simulink model "oculomotor_fb_HW1_2b"  (Simulink 7.8)
settings: Solver=ode45  SolverMode=SingleTasking  StartTime=0.0  StopTime=10  RelTol=1e-3  AbsTol=1e-6
settings Model: Creator=sschaal  LastModifiedBy=okhan  ExtModeAutoUpdateStatusClock=off
settings DataIOCC: LimitDataPoints=off  SaveOutput=off  SaveTime=off  SignalLoggingName=sigsOut
settings OptimizationCC: BooleanDataType=off  InlineInvariantSignals=on  InitFltsAndDblsToZero=on
settings DebuggingCC: SaveWithParameterizedLinksMsg=none  SignalResolutionControl=TryResolveAllWithWarning  SolverPrmCheckMsg=none  MultiTaskDSMMsg=warning  MultiTaskCondExecSysMsg=none  FcnCallInpInsideContextMsg=Use local settings  StrictBusMsg=None
settings HardwareCC: TargetUnknown=on
settings RTWCC: IncludeERTFirstTime=on
settings GRTTargetCC: TargetFcnLib=ansi_tfl_tmw.mat  ModelReferenceCompliant=off  MatFileLogging=off

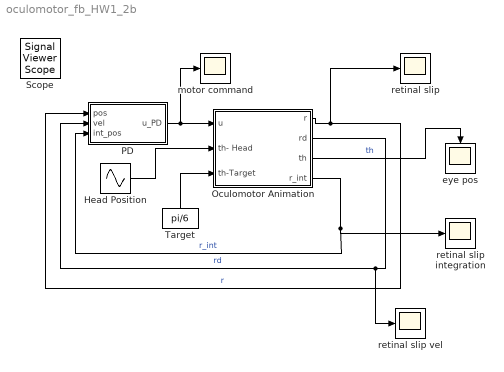
== system oculomotor_fb_HW1_2b ==
  " Target" : Constant  Value=pi/6
  Head Position : Sin  Amplitude=pi/6  Frequency=6  SampleTime=0
  Oculomotor Animation : Subsystem  mask(Oculomotor Animation){ts=0.6, delay=2/60*0.0000001, k=0.4875, b=0.0341, m=3.6889e-4}
      mask prompts: ts "Animation Sampling Time (ts)"; delay "Retinal Slip Delay (delay)"; k "Stiffness (k)"; b "Damping (b)"; m "Mass (m)"
      mask help:
      | Animation Sampling Time: at which freq. to redraw of the animation
      | x-offset: horizontal offset of eye rotation axis from head rotation axis
      | y-offset: vertical offset of eye rotation axis from head rotation axis
      | slip & slip vel. delays: simulated delays for slip computation
      | mass, damping, stiffness: parameters of eye system
      mask Help:
      | Implementation of a second order dynamical model of a 2-eye oculomotor system. Input to the system are the motor commands for left and right eye,
      | the head movement (cause by neck movement or external perturbations), the angle of the visual target (in world coord.), and the foveal length.
      | Outputs are the retinal slip & slip vel. for both eyes and the eye positions.
  PD : Subsystem  mask(PID Controller){P=20, D=0.05, I=1000}
      mask prompts: P "Proportional (P):"; D "Derivative (D):"; I "Integral (I):"
      mask help:
      | Enter expressions for proportional and derivative terms.
      | P+Ds
      mask Help: This block implements a PD controller where parameters are entered for the Proportional and Derivative terms. Unmask this block to see how it works.
  eye pos : Scope
      settings: TickLabels=on  YMin=-0.2  YMax=0.2  DataFormat=Array
  motor command : Scope
      settings: TickLabels=on  YMin=-1  YMax=1  DataFormat=Array
  retinal slip : Scope
      settings: TickLabels=on  TimeRange=10  YMin=0  YMax=0.55  DataFormat=Array
  retinal slip integration : Scope
      settings: TickLabels=on  YMin=-0.2  YMax=0.2  DataFormat=Array
  retinal slip vel : Scope
      settings: TickLabels=on  YMin=-0.2  YMax=0.2  DataFormat=Array
  Scope : SignalViewerScope  IOType=viewer  ZoomMode=xonly  LegendLocations="552.963      402.4925       78.0331      32.50355"  RefreshTime=0.035000
      settings: ShowLegends=on  TimeRange=10  YMin=-0.2  YMax=1.2
  wires:
  " Target"/1 -> Oculomotor Animation/3(th-Target)
  Head Position/1 -> Oculomotor Animation/2(th- Head)
  PD/1(u_PD) -> motor command/1, Oculomotor Animation/1(u)
  Oculomotor Animation/1(r) -> retinal slip/1, PD/1(pos)  "r"
  Oculomotor Animation/2(rd) -> PD/2(vel), retinal slip vel/1  "rd"
  Oculomotor Animation/3(th) -> eye pos/1  "th"
  Oculomotor Animation/4(r_int) -> PD/3(int_pos), retinal slip integration/1  "r_int"

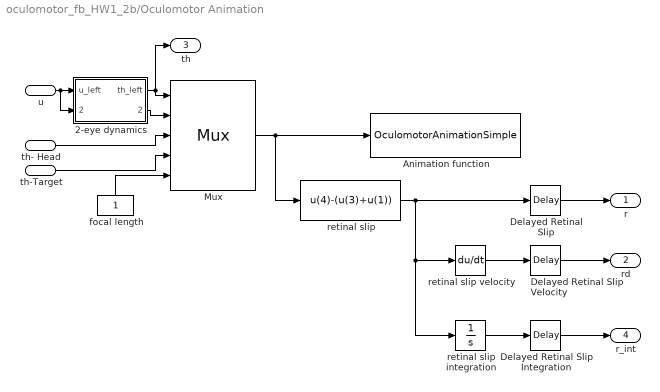
== system oculomotor_fb_HW1_2b/Oculomotor Animation ==
  u : Inport
  th- Head : Inport  Port=2
  th-Target : Inport  Port=3
  " focal length" : Constant
  2-eye dynamics : Subsystem  mask{k=k, b=b, m=m}
      mask prompts: k "Stiffness"; b "Damping"; m "Mass"
  Animation function : S-Function  FunctionName=OculomotorAnimationSimple  Parameters=ts,0,0.1  EnableBusSupport=off
      settings: DeleteFcn=if ~isempty(findobj('type','figure','name','simppend Animation'));close('simppend Animation'); end;
  Delayed Retinal Slip : TransportDelay  DelayTime=delay
  Delayed Retinal Slip Integration : TransportDelay  DelayTime=delay
  Delayed Retinal Slip Velocity : TransportDelay  DelayTime=delay
  Mux : Mux  Inputs=5
      settings: DisplayOption=signals
  retinal slip : Fcn  Expr=u(4)-(u(3)+u(1))
  retinal slip integration : Integrator
  retinal slip velocity : Derivative
  r : Outport
  rd : Outport  Port=2
  th : Outport  Port=3
  r_int : Outport  Port=4
  wires:
  th- Head/1 -> Mux/3
  th-Target/1 -> Mux/4
  Mux/1 -> Animation function/1, retinal slip/1
  2-eye dynamics/1(th_left) -> Mux/1, th/1
  u/1 -> 2-eye dynamics/1(u_left), 2-eye dynamics/2(u_right)
  2-eye dynamics/2(th_right) -> Mux/2
  " focal length"/1 -> Mux/5
  retinal slip/1 -> Delayed Retinal Slip/1, retinal slip velocity/1, retinal slip integration/1
  Delayed Retinal Slip/1 -> r/1
  retinal slip velocity/1 -> Delayed Retinal Slip Velocity/1
  Delayed Retinal Slip Velocity/1 -> rd/1
  retinal slip integration/1 -> Delayed Retinal Slip Integration/1
  Delayed Retinal Slip Integration/1 -> r_int/1

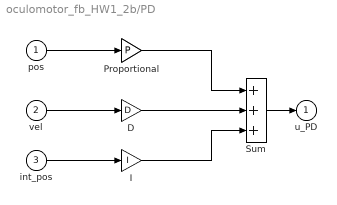
== system oculomotor_fb_HW1_2b/PD ==
  pos : Inport
  vel : Inport  Port=2
  int_pos : Inport  Port=3
  D : Gain  Gain=D  SaturateOnIntegerOverflow=on  OutDataTypeStr=Inherit: Same as input  ParamDataTypeStr=Inherit: Same as input
  I : Gain  Gain=I  SaturateOnIntegerOverflow=on  OutDataTypeStr=Inherit: Same as input  ParamDataTypeStr=Inherit: Same as input
  Proportional : Gain  Gain=P  SaturateOnIntegerOverflow=on  OutDataTypeStr=Inherit: Same as input  ParamDataTypeStr=Inherit: Same as input
  Sum : Sum  Inputs=+++  SaturateOnIntegerOverflow=on  InputSameDT=on  OutDataTypeStr=Inherit: Same as first input
  u_PD : Outport  InitialOutput=0
  wires:
  Sum/1 -> u_PD/1
  Proportional/1 -> Sum/1
  pos/1 -> Proportional/1
  vel/1 -> D/1
  D/1 -> Sum/2
  int_pos/1 -> I/1
  I/1 -> Sum/3

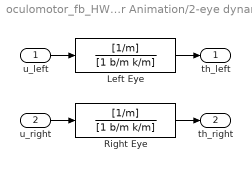
== system oculomotor_fb_HW1_2b/Oculomotor Animation/2-eye dynamics ==
  u_left : Inport
  u_right : Inport  Port=2
  Left Eye : TransferFcn  Numerator=[1/m]  Denominator=[1 b/m k/m]
  Right Eye : TransferFcn  Numerator=[1/m]  Denominator=[1 b/m k/m]
  th_left : Outport  InitialOutput=0
  th_right : Outport  Port=2  InitialOutput=0
  wires:
  u_left/1 -> Left Eye/1
  Left Eye/1 -> th_left/1
  Right Eye/1 -> th_right/1
  u_right/1 -> Right Eye/1
